simulink model "model_troj"  (R2014b)
settings: Solver=ode45  StartTime=0.0  StopTime=10.0  RelTol=1e-3
values from neighbouring files (symbols this model uses):
  k0 = 2    [zad1.m]
  T1 = 3    [zad1.m]
  T2 = 4    [zad1.m]
  troj1_off = troj1_off_tab(i)    [zad1.m]
  troj1_on = troj1_on_tab(i)    [zad1.m]
  troj2_off = troj2_off_tab(i)    [zad1.m]
  troj2_on = troj2_on_tab(i)    [zad1.m]
  zadana = 5    [zad1.m]
settings Model: Creator=Dyzio  LastModifiedBy=Dyzio

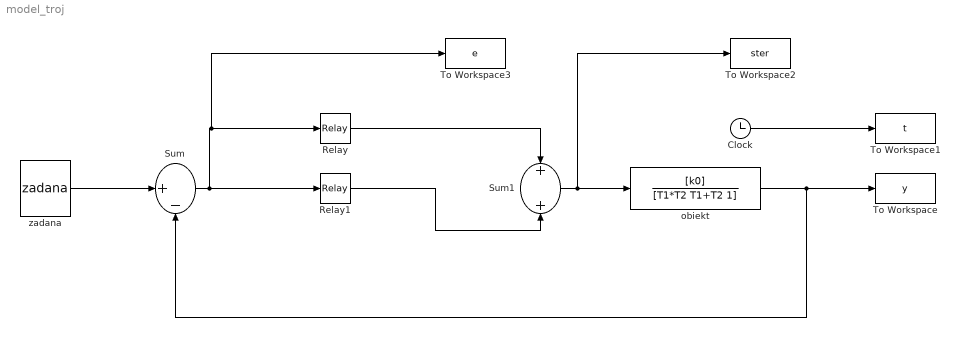
== system model_troj ==
  Clock : Clock
  Relay : Relay  OnSwitchValue=troj1_on  OffSwitchValue=troj1_off  OnOutputValue=zadana  OffOutputValue=-zadana
  Relay1 : Relay  OnSwitchValue=troj2_on  OffSwitchValue=troj2_off  OnOutputValue=zadana  OffOutputValue=-zadana
  Sum : Sum  Inputs=|+-
  Sum1 : Sum  Inputs=+|+
  To Workspace : ToWorkspace  VariableName=y  SampleTime=-1
  To Workspace1 : ToWorkspace  VariableName=t  SampleTime=-1
  To Workspace2 : ToWorkspace  VariableName=ster  SampleTime=-1
  To Workspace3 : ToWorkspace  VariableName=e  SampleTime=-1
  obiekt : TransferFcn  Numerator=[k0]  Denominator=[T1*T2 T1+T2 1]
  zadana : Constant  Value=zadana
  wires:
  zadana/1 -> Sum/1
  obiekt/1 -> Sum/2, To Workspace/1
  Clock/1 -> To Workspace1/1
  Sum/1 -> Relay1/1, Relay/1, To Workspace3/1
  Relay/1 -> Sum1/1
  Relay1/1 -> Sum1/2
  Sum1/1 -> To Workspace2/1, obiekt/1
